simulink model "offline_snac_block"  (R2024a)
settings: Solver=FixedStepAuto  StartTime=0.0  StopTime=inf  RelTol=1e-3  EnableMultiTasking=on
libraries: px4Sensorslib x10, px4uORBlib x3, simulink x2, px4lib x1
settings Model: ExtModeTrigDuration=10  Creator=randy  LastModifiedBy=randy
settings SolverCC: AlgebraicLoopSolver=TrustRegion  PositivePriorityOrder=on  MaxZcPerStep=1
settings OptimizationCC: EnhancedBackFolding=on  PassReuseOutputArgsAs=Individual arguments  ZeroExternalMemoryAtStartup=off  ZeroInternalMemoryAtStartup=off  MaxStackSize=64  OptimizeBlockOrder=speed  DifferentSizesBufferReuse=on  OptimizationCustomize=off  EfficientTunableParamExpr=on
settings DebuggingCC: ParameterTunabilityLossMsg=error  UnconnectedInputMsg=warning  UnconnectedOutputMsg=warning  UnconnectedLineMsg=warning  SymbolicDimsDataTypeCodeGenerationDiagnostic=none
settings HardwareCC: ProdBitPerPointer=32  ProdBitPerSizeT=32  ProdBitPerPtrDiffT=32  ProdLargestAtomicInteger=Long  ProdLargestAtomicFloat=Double  ProdWordSize=32  ProdLongLongMode=on  ProdHWDeviceType=ARM Compatible->ARM Cortex
settings ModelReferenceCC: EnableRefExpFcnMdlSchedulingChecks=on
settings SFSimCC: MATLABDynamicMemAlloc=off  SimTargetLang=C++
settings RTWCC: Description=Embedded Coder  SystemTargetFile=ert.tlc  HardwareBoard=PX4 Cube Orange+  TLCOptions="-aInlineSetEventsForThisBaseRateFcn=TLC_FALSE -aSuppressMultiTaskScheduler=TLC_FALSE  -aRateBasedStepFcn=0"  TemplateMakefile=ert_default_tmf  Toolchain=GNU Tools for PX4 Autopilots  IncludeHyperlinkInReport=on  TargetLang=C++  GPUComputeCapability=3.5  DLArmComputeVersion=19.05
settings CodeAppCC: ForceParamTrailComments=on  IgnoreCustomStorageClasses=off  OperatorAnnotations=on  SimulinkDataObjDesc=on  SFDataObjDesc=on  InsertBlockDesc=on
settings ERTTargetCC: ExtModeTransport=3  ExtModeStaticAlloc=on  ExtModeStaticAllocSize=1024  ExtModeMexFile=ext_xcp  ExtModeIntrfLevel=Level2 - Open

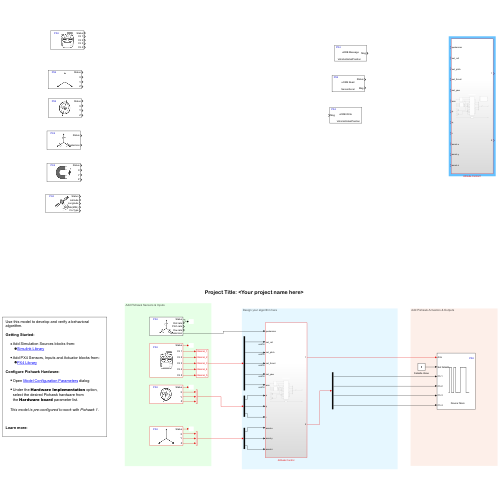
[thumbnail: Simulink's stored preview of the top-level diagram]
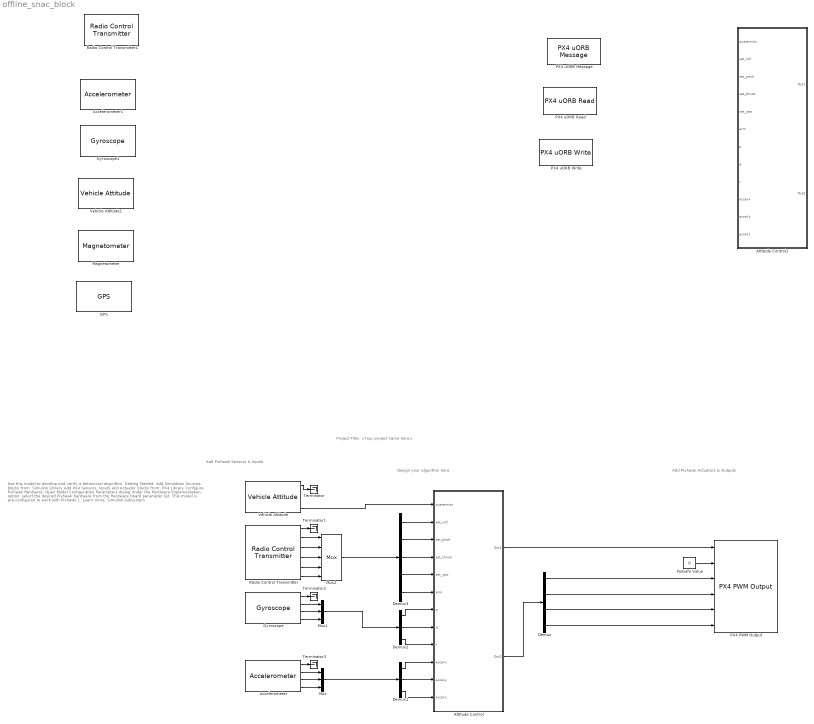
== system offline_snac_block ==
  note: Project Title: <Your project name here>
  note: Use this model to develop and verify a behavioral algorithm.
      |
      | Getting Started:
      |
      | Add Simulation Sources blocks from:
      | Simulink Library
      |
      | Add PX4 Sensors, Inputs and Actuator blocks from:
      | PX4 Library
      |
      | Configure Pixhawk Hardware:
      |
      | Open Model Configuration Parameters dialog
      |
      | Under the Hardware Implementation option, select the desired Pixhawk hardware from the Hardware board parameter list.
      |
      | This model is pre-configured to work with Pixhawk 1.
      |
      | Learn more:
      |
      | Simulink Subsystem
  note: Add Pixhawk Sensors & Inputs
  note: Design your algorithm here
  note: Add Pixhawk Actuators & Outputs
  Accelerometer : px4Sensorslib/Accelerometer  uorbTimeStamp=off  BlockingMode=off  BlockTimeout=1e-3  sampleTime=1/250
  Accelerometer1 : px4Sensorslib/Accelerometer  uorbTimeStamp=off  BlockingMode=off  BlockTimeout=1e-3  sampleTime=1/250
  Attitude Control : Subsystem
  Attitude Control1 : Subsystem
  Demux : Demux
  Demux1 : Demux  Outputs=3
  Demux2 : Demux  Outputs=3
  Demux3 : Demux  Outputs=5
  Failsafe Value : Constant  Value=0  OutDataTypeStr=boolean  SampleTime=-1
  GPS : px4Sensorslib/GPS  lat=on  lon=on  alt=on  velocity=off  course=off  gpsfix=on  numsat=off  timestamp_utc=off  BlockingMode=off  BlockTimeout=1e-3  dop=off  vel_ned=off  alt_ellipsoid=off  jamm_ind=off  timestamp=off  sampleTime=1/250
  Gyroscope : px4Sensorslib/Gyroscope  uorbTimeStamp=off  BlockingMode=off  BlockTimeout=1e-3  sampleTime=1/250
  Gyroscope1 : px4Sensorslib/Gyroscope  uorbTimeStamp=off  BlockingMode=off  BlockTimeout=1e-3  sampleTime=1/250
  Magnetometer : px4Sensorslib/Magnetometer  uorbTimeStamp=off  BlockingMode=off  BlockTimeout=1e-3  sampleTime=1/250
  Mux : Mux  Inputs=3
  Mux1 : Mux  Inputs=3
  Mux2 : Mux  Inputs=5
      settings: DisplayOption=signals
  PX4 PWM Output : px4lib/PX4 PWM Output  pwmDevice=Main  pwmChannel1_=on  pwmChannel2_=on  pwmChannel3_=on  pwmChannel4_=on  pwmChannel5_=off  pwmChannel6_=off  pwmChannel7_=off  pwmChannel8_=off
  PX4 uORB Message : px4uORBlib/PX4 uORB Message  uORBTopic=VehicleGlobalPosition  SampleTime=inf  selectInstance=vehicle_gps_position
  PX4 uORB Read : px4uORBlib/PX4 uORB Read  uORBTopic=SensorAccel  selectInstance=SensorAccel  SampleTime=0.001  BlockingMode=off  BlockTimeout=1e-3
  PX4 uORB Write : px4uORBlib/PX4 uORB Write  uORBTopic=VehicleGlobalPosition  selectInstance=vehicle_gps_position  MessageQueueLen=1
  Radio Control Transmitter : px4Sensorslib/Radio Control Transmitter  channel1=on  channel2=on  channel3=on  channel4=on  channel5=on  channel6=off  channel7=off  channel8=off  channel_count=off  rssi=off  rc_input_source=off  timestamp_last_signal=off  time_stamp=off  sampleTime=1/250  BlockingMode=off  BlockTimeout=5
  Radio Control Transmitter1 : px4Sensorslib/Radio Control Transmitter  channel1=on  channel2=on  channel3=on  channel4=on  channel5=off  channel6=off  channel7=off  channel8=off  channel_count=off  rssi=off  rc_input_source=off  timestamp_last_signal=off  time_stamp=off  sampleTime=1/250  BlockingMode=off  BlockTimeout=5
  Terminator{,1..3} (4 alike) : Terminator
  Vehicle Attitude : px4Sensorslib/Vehicle Attitude  rollRate=on  pitchRate=on  yawRate=on  quaternion=on  uorbTimeStamp=off  BlockingMode=off  BlockTimeout=0.001  sampleTime=1/250
  Vehicle Attitude1 : px4Sensorslib/Vehicle Attitude  rollRate=off  pitchRate=off  yawRate=off  quaternion=on  uorbTimeStamp=off  BlockingMode=off  BlockTimeout=0.001  sampleTime=1/250
  wires:
  Vehicle Attitude/5 -> Attitude Control/1(quaternion)
  Vehicle Attitude/1 -> Terminator/1
  Radio Control Transmitter/1 -> Terminator1/1
  Gyroscope/1 -> Terminator2/1
  Accelerometer/1 -> Terminator3/1
  Failsafe Value/1 -> PX4 PWM Output/2
  Attitude Control/1(Out1) -> PX4 PWM Output/1
  Attitude Control/2(Out2) -> Demux/1
  Demux/4 -> PX4 PWM Output/6
  Demux/3 -> PX4 PWM Output/5
  Demux/2 -> PX4 PWM Output/4
  Demux/1 -> PX4 PWM Output/3
  Accelerometer/3 -> Mux/2
  Accelerometer/2 -> Mux/1
  Accelerometer/4 -> Mux/3
  Mux/1 -> Demux1/1
  Demux1/3 -> Attitude Control/12(accel-z)
  Demux1/2 -> Attitude Control/11(accel-y)
  Demux1/1 -> Attitude Control/10(accel-x)
  Mux1/1 -> Demux2/1
  Gyroscope/2 -> Mux1/1
  Gyroscope/3 -> Mux1/2
  Gyroscope/4 -> Mux1/3
  Demux2/1 -> Attitude Control/7(p)
  Demux2/2 -> Attitude Control/8(q)
  Demux2/3 -> Attitude Control/9(r)
  Mux2/1 -> Demux3/1
  Radio Control Transmitter/2 -> Mux2/1
  Radio Control Transmitter/3 -> Mux2/2
  Radio Control Transmitter/4 -> Mux2/3
  Radio Control Transmitter/5 -> Mux2/4
  Radio Control Transmitter/6 -> Mux2/5
  Demux3/2 -> Attitude Control/3(set_pitch)
  Demux3/3 -> Attitude Control/4(set_thrust)
  Demux3/1 -> Attitude Control/2(set_roll)
  Demux3/4 -> Attitude Control/5(set_yaw)
  Demux3/5 -> Attitude Control/6(arm)

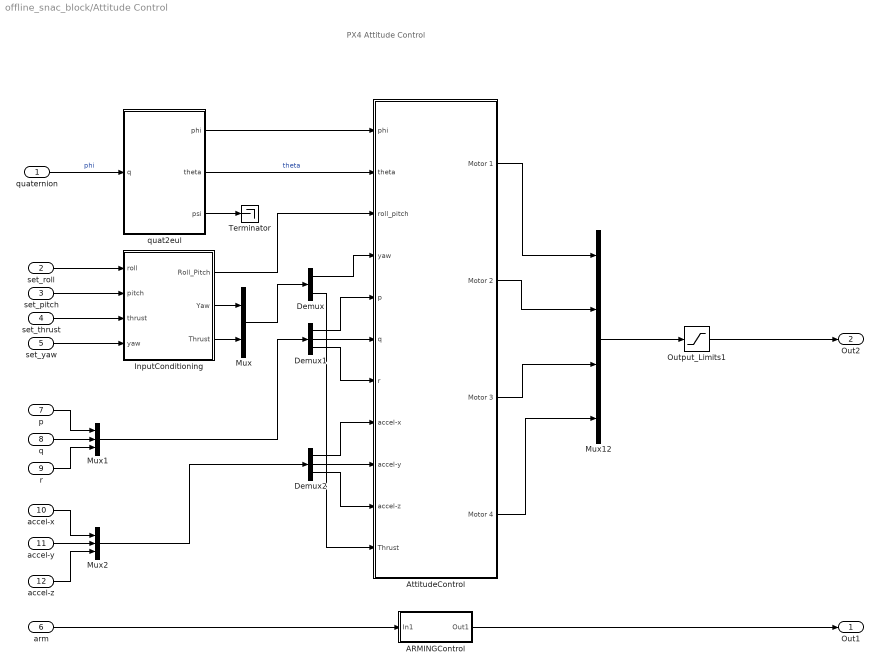
== system offline_snac_block/Attitude Control ==
  note: PX4 Attitude Control
  quaternion : Inport
  set_roll : Inport  Port=2  OutDataTypeStr=uint16
  set_pitch : Inport  Port=3  OutDataTypeStr=uint16
  set_thrust : Inport  Port=4  OutDataTypeStr=uint16
  set_yaw : Inport  Port=5  OutDataTypeStr=uint16
  arm : Inport  Port=6  OutDataTypeStr=uint16
  p : Inport  Port=7
  q : Inport  Port=8
  r : Inport  Port=9
  accel-x : Inport  Port=10
  accel-y : Inport  Port=11
  accel-z : Inport  Port=12
  ARMINGControl : Subsystem
  AttitudeControl : Subsystem
  Demux : Demux  Outputs=2
  Demux1 : Demux  Outputs=3
  Demux2 : Demux  Outputs=3
  InputConditioning : Subsystem
  Mux : Mux  Inputs=2
  Mux1 : Mux  Inputs=3
  Mux12 : Mux
  Mux2 : Mux  Inputs=3
  Output_Limits1 : Saturate  UpperLimit=2000  LowerLimit=1000
  Terminator : Terminator
  quat2eul : MATLAB Function  TreatAsAtomicUnit=on
  Out1 : Outport  VectorParamsAs1DForOutWhenUnconnected=off
  Out2 : Outport  Port=2  VectorParamsAs1DForOutWhenUnconnected=off
  wires:
  set_pitch/1 -> InputConditioning/2(pitch)
  set_roll/1 -> InputConditioning/1(roll)
  arm/1 -> ARMINGControl/1(In1)
  quat2eul/2(theta) -> AttitudeControl/2(theta)  "theta"
  Output_Limits1/1 -> Out2/1
  set_thrust/1 -> InputConditioning/3(thrust)
  Mux12/1 -> Output_Limits1/1
  ARMINGControl/1(Out1) -> Out1/1
  set_yaw/1 -> InputConditioning/4(yaw)
  quaternion/1 -> quat2eul/1(q)  "phi"
  quat2eul/1(phi) -> AttitudeControl/1(phi)
  quat2eul/3(psi) -> Terminator/1
  AttitudeControl/1(Motor 1) -> Mux12/1
  AttitudeControl/2(Motor 2) -> Mux12/2
  AttitudeControl/3(Motor 3) -> Mux12/3
  AttitudeControl/4(Motor 4) -> Mux12/4
  Mux/1 -> Demux/1
  q/1 -> Mux1/2
  p/1 -> Mux1/1
  r/1 -> Mux1/3
  Mux1/1 -> Demux1/1
  Demux1/2 -> AttitudeControl/6(q)
  Demux1/1 -> AttitudeControl/5(p)
  Demux1/3 -> AttitudeControl/7(r)
  accel-y/1 -> Mux2/2
  accel-x/1 -> Mux2/1
  accel-z/1 -> Mux2/3
  Mux2/1 -> Demux2/1
  Demux2/2 -> AttitudeControl/9(accel-y)
  Demux2/1 -> AttitudeControl/8(accel-x)
  Demux2/3 -> AttitudeControl/10(accel-z)
  InputConditioning/2(Yaw) -> Mux/1
  InputConditioning/3(Thrust) -> Mux/2
  InputConditioning/1(Roll_Pitch) -> AttitudeControl/3(roll_pitch)
  Demux/1 -> AttitudeControl/4(yaw)
  Demux/2 -> AttitudeControl/11(Thrust)

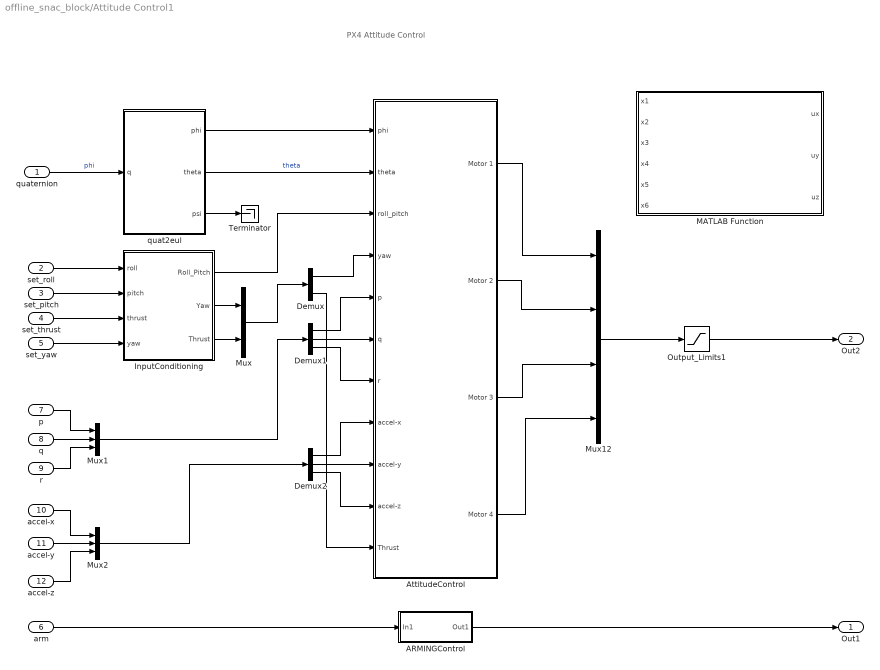
== system offline_snac_block/Attitude Control1 ==
  note: PX4 Attitude Control
  quaternion : Inport
  set_roll : Inport  Port=2  OutDataTypeStr=uint16
  set_pitch : Inport  Port=3  OutDataTypeStr=uint16
  set_thrust : Inport  Port=4  OutDataTypeStr=uint16
  set_yaw : Inport  Port=5  OutDataTypeStr=uint16
  arm : Inport  Port=6  OutDataTypeStr=uint16
  p : Inport  Port=7
  q : Inport  Port=8
  r : Inport  Port=9
  accel-x : Inport  Port=10
  accel-y : Inport  Port=11
  accel-z : Inport  Port=12
  ARMINGControl : Subsystem
  AttitudeControl : Subsystem
  Demux : Demux  Outputs=2
  Demux1 : Demux  Outputs=3
  Demux2 : Demux  Outputs=3
  InputConditioning : Subsystem
  MATLAB Function : MATLAB Function  TreatAsAtomicUnit=on
  Mux : Mux  Inputs=2
  Mux1 : Mux  Inputs=3
  Mux12 : Mux
  Mux2 : Mux  Inputs=3
  Output_Limits1 : Saturate  UpperLimit=2000  LowerLimit=1000
  Terminator : Terminator
  quat2eul : MATLAB Function  TreatAsAtomicUnit=on
  Out1 : Outport  VectorParamsAs1DForOutWhenUnconnected=off
  Out2 : Outport  Port=2  VectorParamsAs1DForOutWhenUnconnected=off
  wires:
  set_pitch/1 -> InputConditioning/2(pitch)
  set_roll/1 -> InputConditioning/1(roll)
  arm/1 -> ARMINGControl/1(In1)
  quat2eul/2(theta) -> AttitudeControl/2(theta)  "theta"
  Output_Limits1/1 -> Out2/1
  set_thrust/1 -> InputConditioning/3(thrust)
  Mux12/1 -> Output_Limits1/1
  ARMINGControl/1(Out1) -> Out1/1
  set_yaw/1 -> InputConditioning/4(yaw)
  quaternion/1 -> quat2eul/1(q)  "phi"
  quat2eul/1(phi) -> AttitudeControl/1(phi)
  quat2eul/3(psi) -> Terminator/1
  AttitudeControl/1(Motor 1) -> Mux12/1
  AttitudeControl/2(Motor 2) -> Mux12/2
  AttitudeControl/3(Motor 3) -> Mux12/3
  AttitudeControl/4(Motor 4) -> Mux12/4
  Mux/1 -> Demux/1
  q/1 -> Mux1/2
  p/1 -> Mux1/1
  r/1 -> Mux1/3
  Mux1/1 -> Demux1/1
  Demux1/2 -> AttitudeControl/6(q)
  Demux1/1 -> AttitudeControl/5(p)
  Demux1/3 -> AttitudeControl/7(r)
  accel-y/1 -> Mux2/2
  accel-x/1 -> Mux2/1
  accel-z/1 -> Mux2/3
  Mux2/1 -> Demux2/1
  Demux2/2 -> AttitudeControl/9(accel-y)
  Demux2/1 -> AttitudeControl/8(accel-x)
  Demux2/3 -> AttitudeControl/10(accel-z)
  InputConditioning/2(Yaw) -> Mux/1
  InputConditioning/3(Thrust) -> Mux/2
  InputConditioning/1(Roll_Pitch) -> AttitudeControl/3(roll_pitch)
  Demux/1 -> AttitudeControl/4(yaw)
  Demux/2 -> AttitudeControl/11(Thrust)

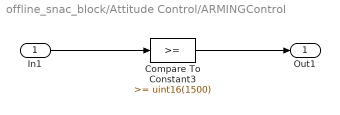
== system offline_snac_block/Attitude Control/ARMINGControl ==
  In1 : Inport
  Compare To Constant3 : simulink/Logic and Bit Operations/Compare To Constant  relop=>=  const=uint16(1500)  OutDataTypeStr=boolean
  Out1 : Outport  VectorParamsAs1DForOutWhenUnconnected=off
  wires:
  Compare To Constant3/1 -> Out1/1
  In1/1 -> Compare To Constant3/1

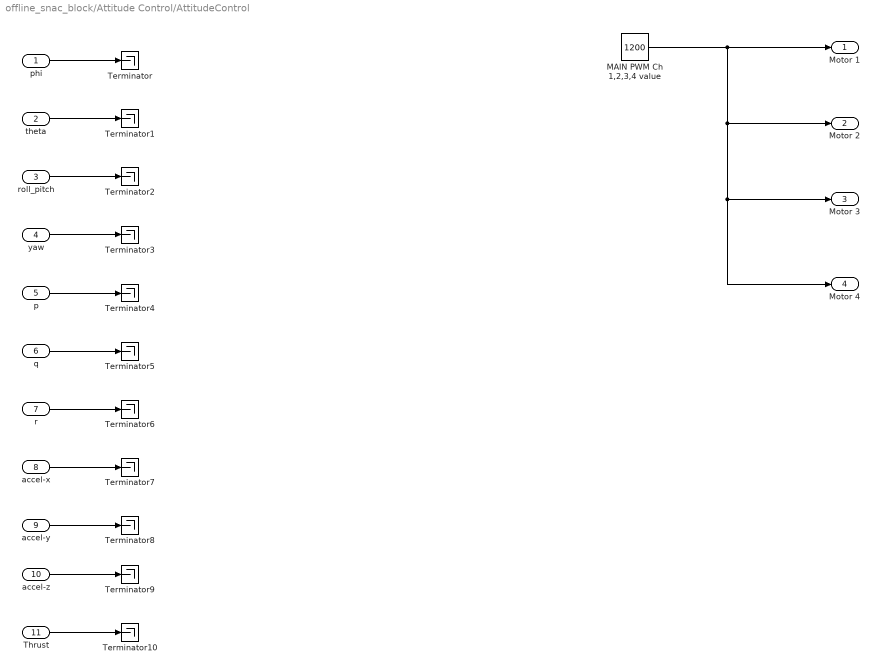
== system offline_snac_block/Attitude Control/AttitudeControl ==
  phi : Inport
  theta : Inport  Port=2
  roll_pitch : Inport  Port=3
  yaw : Inport  Port=4
  p : Inport  Port=5
  q : Inport  Port=6
  r : Inport  Port=7
  accel-x : Inport  Port=8
  accel-y : Inport  Port=9
  accel-z : Inport  Port=10
  Thrust : Inport  Port=11
  MAIN PWM Ch 1,2,3,4 value : Constant  Value=1200  OutDataTypeStr=uint16  SampleTime=1/250
  Terminator{,1..10} (11 alike) : Terminator
  Motor 1 : Outport  OutDataTypeStr=uint16  SampleTime=1/250  VectorParamsAs1DForOutWhenUnconnected=off
  Motor 2 : Outport  Port=2  OutDataTypeStr=uint16  SampleTime=1/250  VectorParamsAs1DForOutWhenUnconnected=off
  Motor 3 : Outport  Port=3  OutDataTypeStr=uint16  SampleTime=1/250  VectorParamsAs1DForOutWhenUnconnected=off
  Motor 4 : Outport  Port=4  OutDataTypeStr=uint16  SampleTime=1/250  VectorParamsAs1DForOutWhenUnconnected=off
  wires:
  phi/1 -> Terminator/1
  theta/1 -> Terminator1/1
  roll_pitch/1 -> Terminator2/1
  yaw/1 -> Terminator3/1
  p/1 -> Terminator4/1
  q/1 -> Terminator5/1
  r/1 -> Terminator6/1
  accel-x/1 -> Terminator7/1
  accel-y/1 -> Terminator8/1
  accel-z/1 -> Terminator9/1
  Thrust/1 -> Terminator10/1
  MAIN PWM Ch 1,2,3,4 value/1 -> Motor 4/1, Motor 3/1, Motor 2/1, Motor 1/1

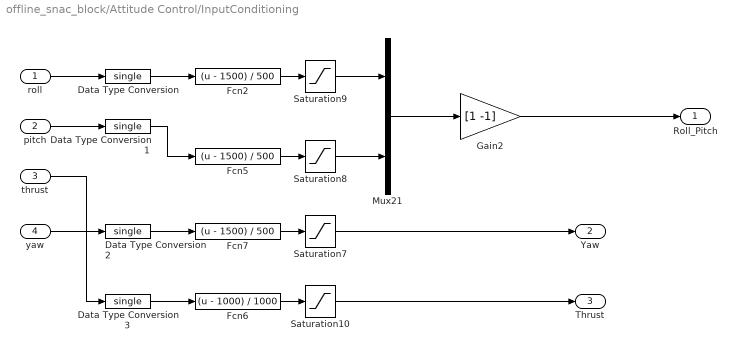
== system offline_snac_block/Attitude Control/InputConditioning ==
  roll : Inport
  pitch : Inport  Port=2
  thrust : Inport  Port=3
  yaw : Inport  Port=4
  Data Type Conversion{,1..3} (4 alike) : DataTypeConversion  OutDataTypeStr=single  SaturateOnIntegerOverflow=off  RndMeth=Floor
  Fcn2 : Fcn  Expr=(u - 1500) / 500
  Fcn5 : Fcn  Expr=(u - 1500) / 500
  Fcn6 : Fcn  Expr=(u - 1000) / 1000
  Fcn7 : Fcn  Expr=(u - 1500) / 500
  Gain2 : Gain  Gain=[1 -1]  OutDataTypeStr=Inherit: Inherit via back propagation
  Mux21 : Mux  Inputs=2
  Saturation10 : Saturate  UpperLimit=1  LowerLimit=0
  Saturation7 : Saturate  UpperLimit=1  LowerLimit=-1
  Saturation8 : Saturate  UpperLimit=1  LowerLimit=-1
  Saturation9 : Saturate  UpperLimit=1  LowerLimit=-1
  Roll_Pitch : Outport  VectorParamsAs1DForOutWhenUnconnected=off
  Yaw : Outport  Port=2  VectorParamsAs1DForOutWhenUnconnected=off
  Thrust : Outport  Port=3  VectorParamsAs1DForOutWhenUnconnected=off
  wires:
  Saturation10/1 -> Thrust/1
  Saturation7/1 -> Yaw/1
  Gain2/1 -> Roll_Pitch/1
  Mux21/1 -> Gain2/1
  Saturation8/1 -> Mux21/2
  Fcn6/1 -> Saturation10/1
  thrust/1 -> Data Type Conversion3/1
  Fcn2/1 -> Saturation9/1
  Fcn5/1 -> Saturation8/1
  Saturation9/1 -> Mux21/1
  Fcn7/1 -> Saturation7/1
  yaw/1 -> Data Type Conversion2/1
  pitch/1 -> Data Type Conversion1/1
  roll/1 -> Data Type Conversion/1
  Data Type Conversion/1 -> Fcn2/1
  Data Type Conversion1/1 -> Fcn5/1
  Data Type Conversion2/1 -> Fcn7/1
  Data Type Conversion3/1 -> Fcn6/1

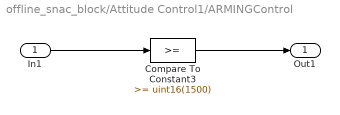
== system offline_snac_block/Attitude Control1/ARMINGControl ==
  In1 : Inport
  Compare To Constant3 : simulink/Logic and Bit Operations/Compare To Constant  relop=>=  const=uint16(1500)  OutDataTypeStr=boolean
  Out1 : Outport  VectorParamsAs1DForOutWhenUnconnected=off
  wires:
  Compare To Constant3/1 -> Out1/1
  In1/1 -> Compare To Constant3/1

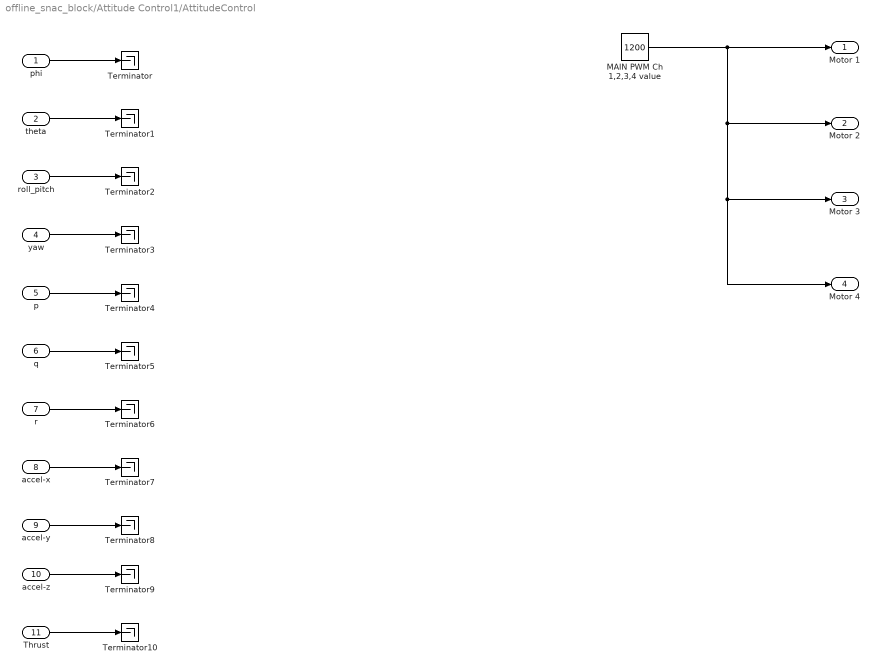
== system offline_snac_block/Attitude Control1/AttitudeControl ==
  phi : Inport
  theta : Inport  Port=2
  roll_pitch : Inport  Port=3
  yaw : Inport  Port=4
  p : Inport  Port=5
  q : Inport  Port=6
  r : Inport  Port=7
  accel-x : Inport  Port=8
  accel-y : Inport  Port=9
  accel-z : Inport  Port=10
  Thrust : Inport  Port=11
  MAIN PWM Ch 1,2,3,4 value : Constant  Value=1200  OutDataTypeStr=uint16  SampleTime=1/250
  Terminator{,1..10} (11 alike) : Terminator
  Motor 1 : Outport  OutDataTypeStr=uint16  SampleTime=1/250  VectorParamsAs1DForOutWhenUnconnected=off
  Motor 2 : Outport  Port=2  OutDataTypeStr=uint16  SampleTime=1/250  VectorParamsAs1DForOutWhenUnconnected=off
  Motor 3 : Outport  Port=3  OutDataTypeStr=uint16  SampleTime=1/250  VectorParamsAs1DForOutWhenUnconnected=off
  Motor 4 : Outport  Port=4  OutDataTypeStr=uint16  SampleTime=1/250  VectorParamsAs1DForOutWhenUnconnected=off
  wires:
  phi/1 -> Terminator/1
  theta/1 -> Terminator1/1
  roll_pitch/1 -> Terminator2/1
  yaw/1 -> Terminator3/1
  p/1 -> Terminator4/1
  q/1 -> Terminator5/1
  r/1 -> Terminator6/1
  accel-x/1 -> Terminator7/1
  accel-y/1 -> Terminator8/1
  accel-z/1 -> Terminator9/1
  Thrust/1 -> Terminator10/1
  MAIN PWM Ch 1,2,3,4 value/1 -> Motor 4/1, Motor 3/1, Motor 2/1, Motor 1/1

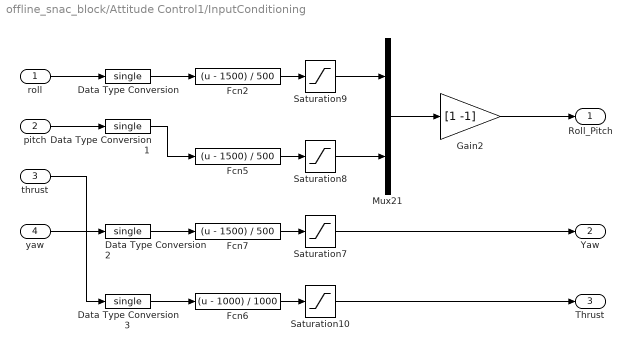
== system offline_snac_block/Attitude Control1/InputConditioning ==
  roll : Inport
  pitch : Inport  Port=2
  thrust : Inport  Port=3
  yaw : Inport  Port=4
  Data Type Conversion{,1..3} (4 alike) : DataTypeConversion  OutDataTypeStr=single  SaturateOnIntegerOverflow=off  RndMeth=Floor
  Fcn2 : Fcn  Expr=(u - 1500) / 500
  Fcn5 : Fcn  Expr=(u - 1500) / 500
  Fcn6 : Fcn  Expr=(u - 1000) / 1000
  Fcn7 : Fcn  Expr=(u - 1500) / 500
  Gain2 : Gain  Gain=[1 -1]  OutDataTypeStr=Inherit: Inherit via back propagation
  Mux21 : Mux  Inputs=2
  Saturation10 : Saturate  UpperLimit=1  LowerLimit=0
  Saturation7 : Saturate  UpperLimit=1  LowerLimit=-1
  Saturation8 : Saturate  UpperLimit=1  LowerLimit=-1
  Saturation9 : Saturate  UpperLimit=1  LowerLimit=-1
  Roll_Pitch : Outport  VectorParamsAs1DForOutWhenUnconnected=off
  Yaw : Outport  Port=2  VectorParamsAs1DForOutWhenUnconnected=off
  Thrust : Outport  Port=3  VectorParamsAs1DForOutWhenUnconnected=off
  wires:
  Saturation10/1 -> Thrust/1
  Saturation7/1 -> Yaw/1
  Gain2/1 -> Roll_Pitch/1
  Mux21/1 -> Gain2/1
  Saturation8/1 -> Mux21/2
  Fcn6/1 -> Saturation10/1
  thrust/1 -> Data Type Conversion3/1
  Fcn2/1 -> Saturation9/1
  Fcn5/1 -> Saturation8/1
  Saturation9/1 -> Mux21/1
  Fcn7/1 -> Saturation7/1
  yaw/1 -> Data Type Conversion2/1
  pitch/1 -> Data Type Conversion1/1
  roll/1 -> Data Type Conversion/1
  Data Type Conversion/1 -> Fcn2/1
  Data Type Conversion1/1 -> Fcn5/1
  Data Type Conversion2/1 -> Fcn7/1
  Data Type Conversion3/1 -> Fcn6/1

== matlab function offline_snac_block/Attitude Control1/quat2eul ==
  data: q input; phi output; theta output; psi output
function [phi,theta,psi] = quat2eul(q)

% Quaternion conversion to Euler angles based on the PX4 Firmware v1.6.5
% release.

phi = atan2(2*(q(1)*q(2) + q(3)* q(4)), q(1)^2 - q(2)^2 - q(3)^2 + q(4)^2);
theta = asin(-2*(q(2)*q(4) - q(1)*q(3)));
psi = atan2(2*(q(2)*q(3) + q(1)* q(4)), q(1)^2 + q(2)^2 - q(3)^2 - q(4)^2);

end

== matlab function offline_snac_block/Attitude Control1/MATLAB Function ==
  data: x1 input; ux output; x2 input; uy output; x3 input; x4 input; x5 input; x6 input; uz output
function [ux, uy, uz] = pos_controller(x1, x2, x3, x4, x5, x6)
    
    % Position_Q = dt*diag([1e6,1e6,1e5,1e5,1e5,1e5]);

    Position_R = dt*diag([0.5e4,0.5e4,0.5e4]);
    uXYZ = -Position_R^-1 * Position_G(x(1:6,i)-r_smooth(:, i))' * Position_W(:,:)' * Basis_Func_84(x(1:6,i)-r_smooth(:, i));

    ux = uXYZ(1);
    uy = uXYZ(2);
    uz = uXYZ(3);
end

== matlab function offline_snac_block/Attitude Control/quat2eul ==
  data: q input; phi output; theta output; psi output
function [phi,theta,psi] = quat2eul(q)

% Quaternion conversion to Euler angles based on the PX4 Firmware v1.6.5
% release.

phi = atan2(2*(q(1)*q(2) + q(3)* q(4)), q(1)^2 - q(2)^2 - q(3)^2 + q(4)^2);
theta = asin(-2*(q(2)*q(4) - q(1)*q(3)));
psi = atan2(2*(q(2)*q(3) + q(1)* q(4)), q(1)^2 + q(2)^2 - q(3)^2 - q(4)^2);

end
